simulink model "P_SP_models"  (R2021a)
settings: Solver=VariableStepAuto  StartTime=0.0  StopTime=30  MaxStep=0.0001  RelTol=1e-3
model workspace (MAT data in the model file):
  am = 1
libraries: simulink x1
settings Model: Creator=valerio  LastModifiedBy=simon
settings SolverCC: AlgebraicLoopSolver=TrustRegion
settings DebuggingCC: SFMachineParentedDataDiag=warning

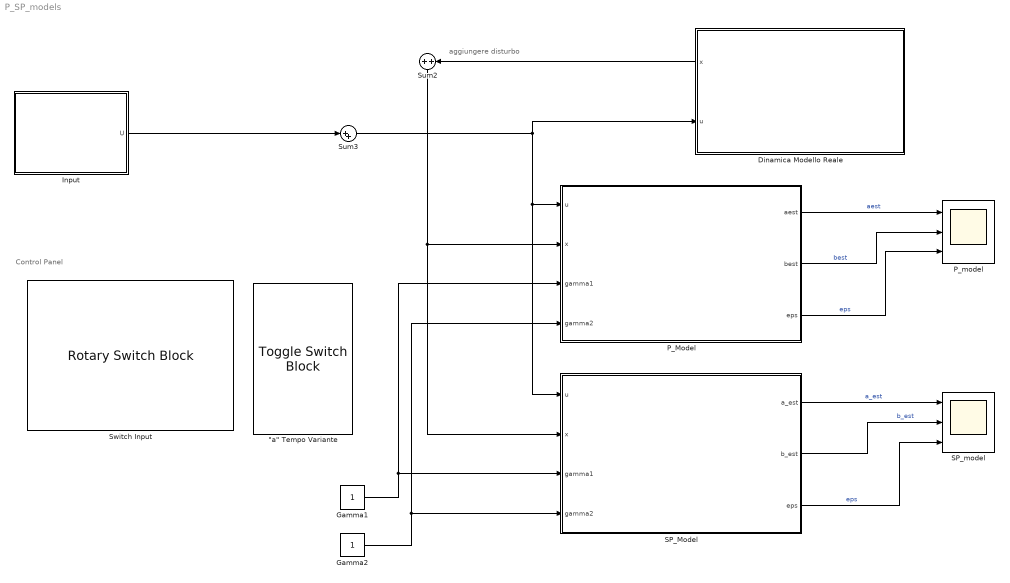
== system P_SP_models ==
  note: Control Panel
  note: aggiungere disturbo
  " \"a\" Tempo Variante" : ToggleSwitchBlock  LabelPosition=Hide
      settings: Values={{'Off', 'On'}, [1 2]}
  Dinamica Modello Reale : Subsystem
      settings: PortSchema="{\"entries\":[{\"content\":{\"sides\":[{\"content\":{\"connectorIds\":[\"Out1\",\"In1\"]},\"type\":\"ConnectorPlacement.EquallySpacedRectSide\",\"uuid\":\"29482476-401b-41e7-9ad6-c6af3f7ca46f\"},{\"content\":{\"connectorIds\":[],\"side\":\"RIGHT\"},\"type\":\"ConnectorPlacement.EquallySpacedRectSide\",\"uuid\":\"f6eae66b-0fdb-4798-98ce-b6245a6528d3\"},{\"content\":{\"connectorIds\":[],\"side\":\"TOP\"},\"type\":\"ConnectorPlacement.EquallySpacedRectSide\",\"uuid\":\"bf44f428-fe33-46a7-93c0-690038f41b99\"}]},\"type\":\"ConnectorPlacement.EquallySpacedConnector\",\"uuid\":\"07e71849-cf32-484a-a28b-980fa66d4ee9\"}],\"packageUris\":[\"http://schema.mathworks.com/mf0/Connector/R2020b\"],\"version\":\"1.0\"}"
  Gamma1 : Constant
  Gamma2 : Constant
  Input : Subsystem
  P_Model : Subsystem
  P_model : Scope  NumInputPorts=3
  SP_Model : Subsystem
  SP_model : Scope  NumInputPorts=3
  Sum2 : Sum  Inputs=+|+
  Sum3 : Sum  Inputs=|++
  Switch Input : RotarySwitchBlock  LabelPosition=Hide
      settings: Values={{'sin', 'step', 'ramp'}, [1 2 3]}
  wires:
  Sum3/1 -> SP_Model/1(u), P_Model/1(u), Dinamica Modello Reale/1(u)
  Dinamica Modello Reale/1(x) -> Sum2/2
  Input/1(U) -> Sum3/1
  Sum2/1 -> SP_Model/2(x), P_Model/2(x)
  P_Model/1(aest) -> P_model/1  "aest"
  P_Model/2(best) -> P_model/2  "best"
  P_Model/3(eps) -> P_model/3  "eps"
  SP_Model/3(eps) -> SP_model/3  "eps"
  SP_Model/1(a_est) -> SP_model/1  "a_est"
  SP_Model/2(b_est) -> SP_model/2  "b_est"
  Gamma1/1 -> SP_Model/3(gamma1), P_Model/3(gamma1)
  Gamma2/1 -> SP_Model/4(gamma2), P_Model/4(gamma2)

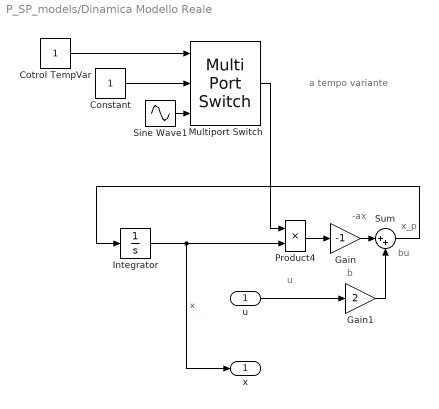
== system P_SP_models/Dinamica Modello Reale ==
  note: a tempo variante
  note: b
  note: bu
  note: -ax
  note: x_p
  note: u
  u : Inport
  Constant : Constant
  Cotrol TempVar : Constant
  Gain : Gain  Gain=-1
  Gain1 : Gain  Gain=2
  Integrator : Integrator
  Multiport Switch : MultiPortSwitch  Inputs=2
  Product4 : Product
  Sine Wave1 : Sin  Bias=1  Frequency=2*pi/(24*3600)  SampleTime=0
  Sum : Sum  Inputs=|++
  x : Outport
  wires:
  Gain/1 -> Sum/1
  Sum/1 -> Integrator/1
  Gain1/1 -> Sum/2
  Integrator/1 -> Product4/2, x/1  "x"
  u/1 -> Gain1/1
  Product4/1 -> Gain/1
  Multiport Switch/1 -> Product4/1
  Cotrol TempVar/1 -> Multiport Switch/1
  Constant/1 -> Multiport Switch/2
  Sine Wave1/1 -> Multiport Switch/3

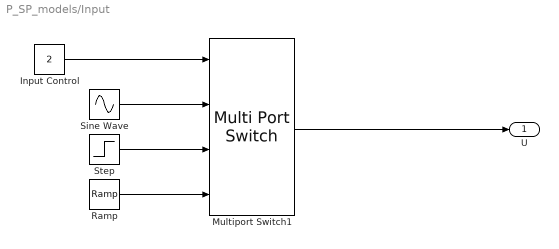
== system P_SP_models/Input ==
  Input Control : Constant  Value=2
  Multiport Switch1 : MultiPortSwitch
  Ramp : simulink/Sources/Ramp  slope=1  start=0  InitialOutput=0
  Sine Wave : Sin  SampleTime=0
  Step : Step  Time=0  SampleTime=0
  U : Outport
  wires:
  Input Control/1 -> Multiport Switch1/1
  Ramp/1 -> Multiport Switch1/4
  Sine Wave/1 -> Multiport Switch1/2
  Multiport Switch1/1 -> U/1
  Step/1 -> Multiport Switch1/3

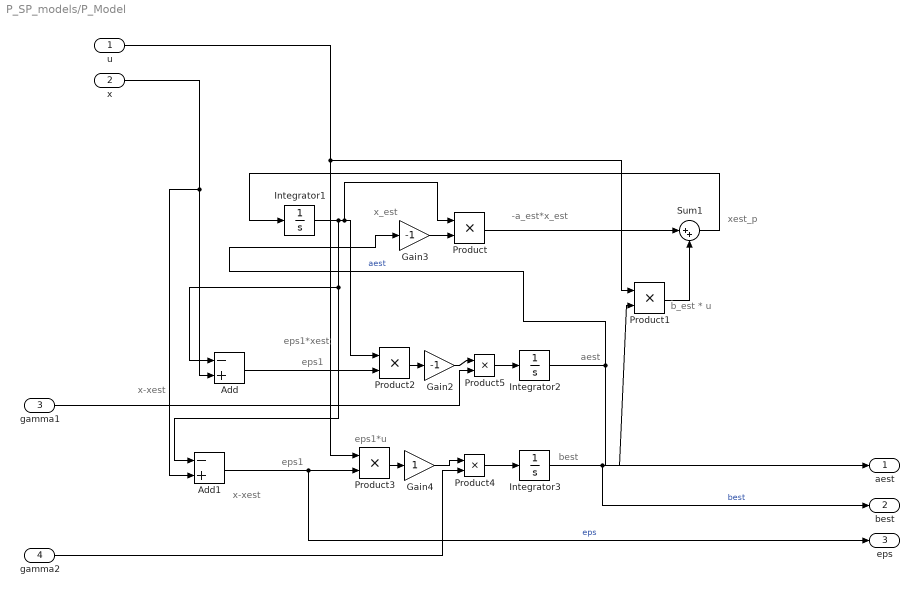
== system P_SP_models/P_Model ==
  note: eps1*xest
  note: eps1*u
  note: x-xest
  note: eps1
  note: eps1
  note: best
  note: aest
  note: x_est
  note: -a_est*x_est
  note: b_est * u
  note: xest_p
  note: x-xest
  u : Inport
  x : Inport  Port=2
  gamma1 : Inport  Port=3
  gamma2 : Inport  Port=4
  Add : Sum  Inputs=-+
  Add1 : Sum  Inputs=-+
  Gain2 : Gain  Gain=-1
  Gain3 : Gain  Gain=-1
  Gain4 : Gain
  Integrator1 : Integrator
  Integrator2 : Integrator
  Integrator3 : Integrator
  Product{,1..5} (6 alike) : Product
  Sum1 : Sum  Inputs=|++
  aest : Outport
  best : Outport  Port=2
  eps : Outport  Port=3
  wires:
  Product1/1 -> Sum1/2
  Product2/1 -> Gain2/1
  Product/1 -> Sum1/1
  Integrator1/1 -> Add1/1, Add/1, Product2/1, Product/1
  x/1 -> Add1/2, Add/2
  Add/1 -> Product2/2
  Add1/1 -> eps/1, Product3/2  "eps"
  Integrator2/1 -> aest/1, Gain3/1  "aest"
  u/1 -> Product1/1, Product3/1
  Integrator3/1 -> best/1, Product1/2  "best"
  Gain3/1 -> Product/2
  Sum1/1 -> Integrator1/1
  Product3/1 -> Gain4/1
  Product5/1 -> Integrator2/1
  Gain2/1 -> Product5/1
  Product4/1 -> Integrator3/1
  Gain4/1 -> Product4/1
  gamma2/1 -> Product4/2
  gamma1/1 -> Product5/2

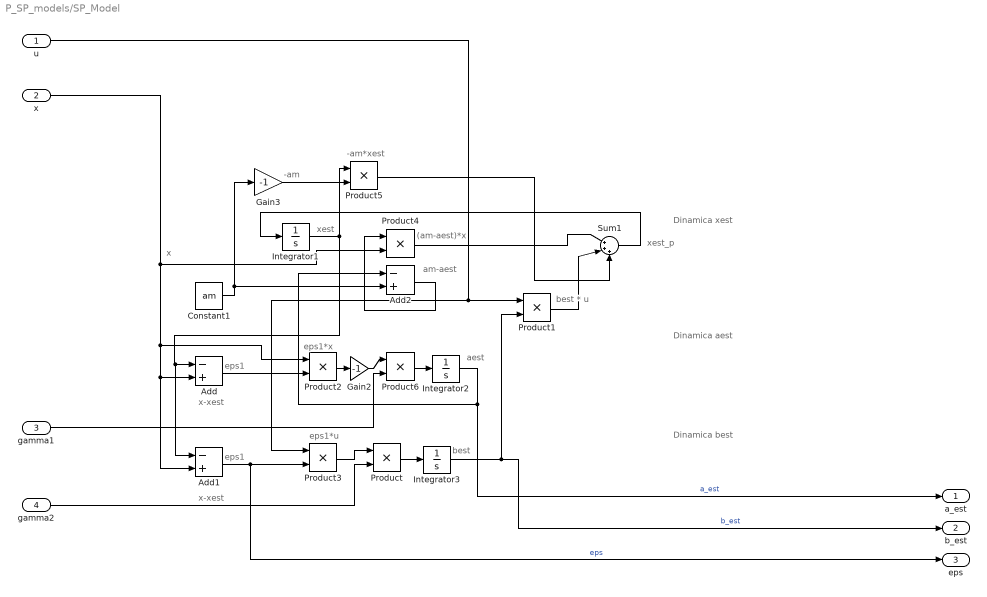
== system P_SP_models/SP_Model ==
  note: -am*xest
  note: -am
  note: (am-aest)*x
  note: am-aest
  note: x
  note: xest
  note: best * u
  note: Dinamica xest
  note: xest_p
  note: x-xest
  note: x-xest
  note: eps1*u
  note: eps1*x
  note: Dinamica aest
  note: aest
  note: Dinamica best
  note: best
  note: eps1
  note: eps1
  u : Inport
  x : Inport  Port=2
  gamma1 : Inport  Port=3
  gamma2 : Inport  Port=4
  Add : Sum  Inputs=-+
  Add1 : Sum  Inputs=-+
  Add2 : Sum  Inputs=-+
  Constant1 : Constant  Value=am
  Gain2 : Gain  Gain=-1
  Gain3 : Gain  Gain=-1
  Integrator1 : Integrator
  Integrator2 : Integrator
  Integrator3 : Integrator
  Product{,1..6} (7 alike) : Product
  Sum1 : Sum  Inputs=|+++
  a_est : Outport
  b_est : Outport  Port=2
  eps : Outport  Port=3
  wires:
  Constant1/1 -> Gain3/1, Add2/2
  Add1/1 -> eps/1, Product3/2  "eps"
  Integrator2/1 -> Add2/1, a_est/1  "a_est"
  Integrator1/1 -> Product5/1, Add1/1, Add/1
  Integrator3/1 -> b_est/1, Product1/2  "b_est"
  Sum1/1 -> Integrator1/1
  u/1 -> Product3/1, Product1/1
  Add/1 -> Product2/2
  Add2/1 -> Product4/1
  Product3/1 -> Product/1
  x/1 -> Product4/2, Add1/2, Add/2, Product2/1
  Product1/1 -> Sum1/2
  Gain3/1 -> Product5/2
  Product5/1 -> Sum1/3
  Product4/1 -> Sum1/1
  Product2/1 -> Gain2/1
  gamma2/1 -> Product/2
  Product6/1 -> Integrator2/1
  Gain2/1 -> Product6/1
  gamma1/1 -> Product6/2
  Product/1 -> Integrator3/1
